simulink model "quadratur_mod1"  (Simulink 6.1)
settings: Solver=ode45  StartTime=0.0  StopTime=10.0  RelTol=1e-3
values from neighbouring files (symbols this model uses):
  f1 = 0.1    [CFIR_1.m]    (also in analog_bp1.m = ',num2str(f1),' Hz; analog_bp11.m = ',num2str(f1),' Hz; analog_bp2.m = 30000; analog_bp3.m = 30000)
  f2 = 0.3    [CFIR_1.m]    (also in analog_bp1.m = ',num2str(f2),' Hz)']); analog_bp11.m = ',num2str(f2),' Hz)']); analog_bp2.m = 35000; analog_bp3.m = 30500)
  fs = 16000    [G722_1.m]    (also in TP_fdesign1.m = 0.215; adaptiv_2.m = 1000; adaptiv_3.m = 1000; adaptiv_4.m = 1000)
undefined symbols (not defined in the file or in its folder): bc_i, bc_r, f0, fs0, get, h_bp
libraries: dsparch4 x3, dspsnks4 x2
settings Model: Creator=svenhoffmann  LastModifiedBy=svenhoffmann  ExtModeAutoUpdateStatusClock=off
settings DataIOCC: LimitDataPoints=off  MaxDataPoints=1  SignalLoggingName=sigsOut
settings HardwareCC: TargetUnknown=on

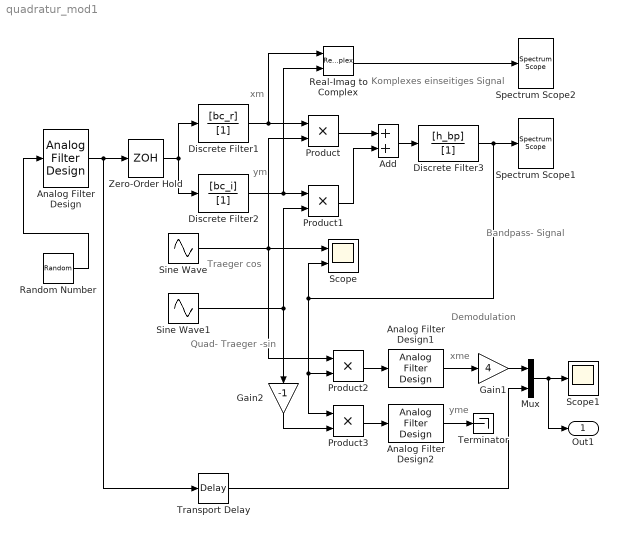
== system quadratur_mod1 ==
  note: xm
  note: ym
  note: Demodulation
  note: xme
  note: yme
  note: Komplexes einseitiges
      | Signal
  note: Bandpass-
      | Signal
  note: Traeger
      | cos
  note: Quad-
      | Traeger
      | -sin
  Add : Sum  OutScaling=2^-10
  Analog Filter Design : dsparch4/Analog Filter Design  method=Chebyshev I  filttype=Bandpass  N=8  Wlo=2*pi*f1  Whi=2*pi*f2  Rp=2  Rs=40
  Analog Filter Design1 : dsparch4/Analog Filter Design  method=Butterworth  filttype=Lowpass  N=8  Wlo=2*pi*300  Whi=80  Rp=2  Rs=40
  Analog Filter Design2 : dsparch4/Analog Filter Design  method=Butterworth  filttype=Lowpass  N=8  Wlo=2*pi*300  Whi=80  Rp=2  Rs=40
  Discrete Filter1 : DiscreteFilter  Numerator=[bc_r]  Denominator=[1]  SampleTime=1/fs
  Discrete Filter2 : DiscreteFilter  Numerator=[bc_i]  Denominator=[1]  SampleTime=1/fs
  Discrete Filter3 : DiscreteFilter  Numerator=[h_bp]  Denominator=[1]  SampleTime=1/fs0
  Gain1 : Gain  Gain=4
  Gain2 : Gain  Orientation=down  Gain=-1
  Mux : Mux  Inputs=2
  Product{,1..3} (4 alike) : Product  RndMeth=Zero
  Random Number : RandomNumber  SampleTime=0
  Real-Imag to Complex : RealImagToComplex
  Scope : Scope  NumInputPorts=2
      settings: YMin=-5~-5  YMax=5~5
  Scope1 : Scope
  Sine Wave : Sin  Frequency=2*pi*f0  SampleTime=1/fs0
  Sine Wave1 : Sin  Frequency=2*pi*f0  Phase=pi/2  SampleTime=1/fs0
  Spectrum Scope1 : dspsnks4/Spectrum Scope  ScopeProperties=off  Domain=Frequency  HorizSpan=1  UseBuffer=on  BufferSize=256  Overlap=64  inpFftLenInherit=on  FFTlength=256  numAvg=20  DisplayProperties=on  AxisGrid=on  Memory=off  FrameNumber=on  AxisLegend=off  AxisZoom=off  OpenScopeAtSimStart=on  OpenScopeImmediately=off  FigPos=get(0,'defaultfigureposition')  AxisProperties=off  XUnits=Hertz  XRange=[0...Fs]  InheritXIncr=on  XIncr=1.0  XLabel=Samples  YUnits=dB  YLabel=Magnitude, dB  LineProperties=off  wintypeSpecScope=Hann  RsSpecScope=50  betaSpecScope=5  winsampSpecScope=Periodic
      settings: YMin=-164.362377632534  YMax=15.8101220793404
  Spectrum Scope2 : dspsnks4/Spectrum Scope  ScopeProperties=off  Domain=Frequency  HorizSpan=1  UseBuffer=on  BufferSize=256  Overlap=64  inpFftLenInherit=on  FFTlength=256  numAvg=20  DisplayProperties=on  AxisGrid=on  Memory=off  FrameNumber=on  AxisLegend=off  AxisZoom=off  OpenScopeAtSimStart=on  OpenScopeImmediately=off  FigPos=get(0,'defaultfigureposition')  AxisProperties=off  XUnits=Hertz  XRange=[0...Fs]  InheritXIncr=on  XIncr=1.0  XLabel=Samples  YUnits=dB  YLabel=Magnitude, dB  LineProperties=off  wintypeSpecScope=Hann  RsSpecScope=50  betaSpecScope=5  winsampSpecScope=Periodic
      settings: YMin=-164.362377632534  YMax=15.8101220793404
  Terminator : Terminator
  Transport Delay : TransportDelay  DelayTime=0.057
  Zero-Order Hold : ZeroOrderHold  SampleTime=1/fs
  Out1 : Outport
  wires:
  Analog Filter Design/1 -> Zero-Order Hold/1, Transport Delay/1
  Zero-Order Hold/1 -> Discrete Filter2/1, Discrete Filter1/1
  Random Number/1 -> Analog Filter Design/1
  Discrete Filter1/1 -> Product/1, Real-Imag to Complex/1
  Discrete Filter2/1 -> Product1/1, Real-Imag to Complex/2
  Sine Wave/1 -> Product/2, Scope/1, Product2/1
  Sine Wave1/1 -> Product1/2, Gain2/1
  Product/1 -> Add/1
  Product1/1 -> Add/2
  Add/1 -> Discrete Filter3/1
  Discrete Filter3/1 -> Spectrum Scope1/1, Scope/2, Product2/2, Product3/1
  Product2/1 -> Analog Filter Design1/1
  Real-Imag to Complex/1 -> Spectrum Scope2/1
  Analog Filter Design1/1 -> Gain1/1
  Mux/1 -> Scope1/1, Out1/1
  Transport Delay/1 -> Mux/2
  Gain1/1 -> Mux/1
  Product3/1 -> Analog Filter Design2/1
  Gain2/1 -> Product3/2
  Analog Filter Design2/1 -> Terminator/1
